simulink model "pid_position1"  (R2016b)
settings: Solver=VariableStepAuto  StartTime=0.0  StopTime=1  RelTol=1e-3
values from neighbouring files (symbols this model uses):
  Kd = -(1/(num(2,3)+num(2,4))*(poles(1)+poles(2)+poles(3))+den(1,2)/(num(2,3)+num(2,4)))*pi/180    [position1.m]    (also in position2.m = (1/(num(2,3)+num(2,4))*(poles(1)+poles(2)+poles(3))+den(1,2))
  Kd_p = 0    [position1.m]    (also in position2.m = 4.87)
  Ki = -(1/(num(2,3)+num(2,4))*(poles(1)*poles(2)*poles(3))+den(1,4)/(num(2,3)+num(2,4)))*pi/180    [position1.m]    (also in position2.m = (1/(num(2,3)+num(2,4))*(poles(1)*poles(2)*poles(3))+den(1,4))
  Ki_p = 0    [position1.m]    (also in position2.m = 0.197)
  Kp = -(den(1,3)/(num(2,3)+num(2,4))-1/(num(2,3)+num(2,4))*(poles(1)*poles(2)+poles(1)*poles(3)+poles(2)*poles(3)))*pi/180    [position1.m]    (also in position2.m = (den(1,3)/(num(2,3)+num(2,4))-1/(num(2,3)+num(2,4))*(poles(1)
  Kp_p = 16.8    [position1.m]    (also in position2.m = 1.96)
undefined symbols (not defined in the file or in its folder): den, num
settings Model: Creator=Ernie  LastModifiedBy=Ernie

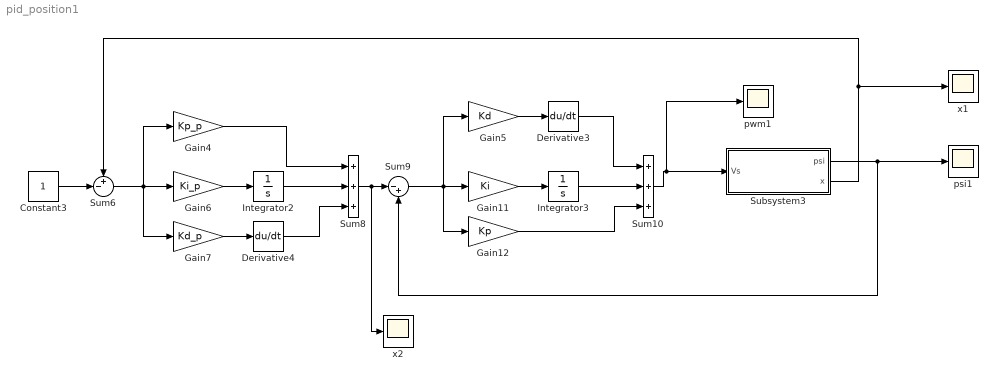
== system pid_position1 ==
  Constant3 : Constant
  Derivative3 : Derivative
  Derivative4 : Derivative
  Gain11 : Gain  Gain=Ki
  Gain12 : Gain  Gain=Kp
  Gain4 : Gain  Gain=Kp_p
  Gain5 : Gain  Gain=Kd
  Gain6 : Gain  Gain=Ki_p
  Gain7 : Gain  Gain=Kd_p
  Integrator2 : Integrator
  Integrator3 : Integrator
  Subsystem3 : Subsystem
  Sum10 : Sum  Inputs=+++
  Sum6 : Sum  Inputs=+-|
  Sum8 : Sum  Inputs=+++
  Sum9 : Sum  Inputs=|-+
  psi1 : Scope
  pwm1 : Scope
  x1 : Scope
  x2 : Scope
  wires:
  Sum8/1 -> x2/1, Sum9/1
  Gain11/1 -> Integrator3/1
  Integrator3/1 -> Sum10/2
  Gain12/1 -> Sum10/3
  Derivative3/1 -> Sum10/1
  Gain5/1 -> Derivative3/1
  Sum9/1 -> Gain5/1, Gain12/1, Gain11/1
  Subsystem3/1(psi) -> psi1/1, Sum9/2
  Constant3/1 -> Sum6/2
  Subsystem3/2(x) -> Sum6/1, x1/1
  Sum6/1 -> Gain7/1, Gain6/1, Gain4/1
  Gain7/1 -> Derivative4/1
  Gain6/1 -> Integrator2/1
  Derivative4/1 -> Sum8/3
  Integrator2/1 -> Sum8/2
  Gain4/1 -> Sum8/1
  Sum10/1 -> Subsystem3/1(Vs), pwm1/1

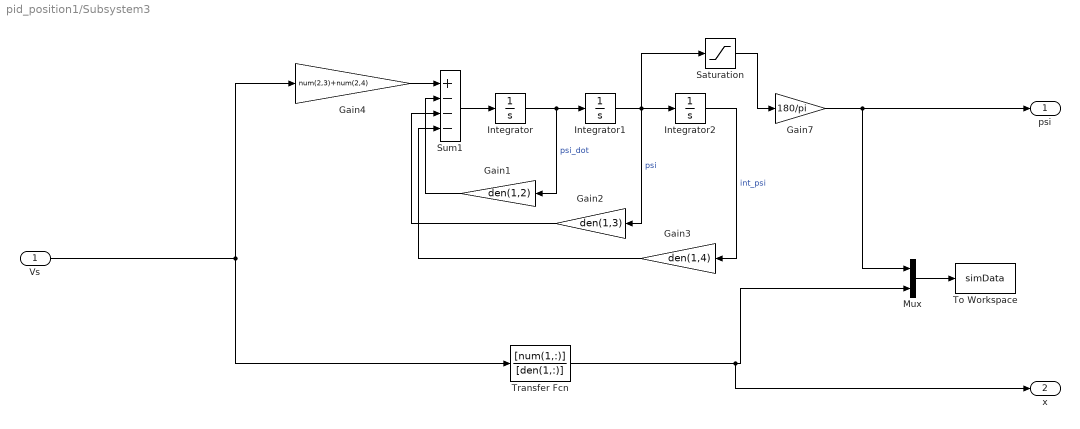
== system pid_position1/Subsystem3 ==
  Vs : Inport
  Gain1 : Gain  Gain=den(1,2)
  Gain2 : Gain  Gain=den(1,3)
  Gain3 : Gain  Gain=den(1,4)
  Gain4 : Gain  Gain=num(2,3)+num(2,4)
  Gain7 : Gain  Gain=180/pi
  Integrator : Integrator
  Integrator1 : Integrator  InitialCondition=10*pi/180
  Integrator2 : Integrator
  Mux : Mux  Inputs=2
  Saturation : Saturate  UpperLimit=pi/2  LowerLimit=-pi/2
  Sum1 : Sum  Inputs=+---
  To Workspace : ToWorkspace  VariableName=simData  SaveFormat=Timeseries  SampleTime=-1
  Transfer Fcn : TransferFcn  Numerator=[num(1,:)]  Denominator=[den(1,:)]
  psi : Outport
  x : Outport  Port=2
  wires:
  Mux/1 -> To Workspace/1
  Gain7/1 -> Mux/1, psi/1
  Integrator/1 -> Gain1/1, Integrator1/1  "psi_dot"
  Integrator1/1 -> Saturation/1, Gain2/1, Integrator2/1  "psi"
  Sum1/1 -> Integrator/1
  Gain1/1 -> Sum1/2
  Gain2/1 -> Sum1/3
  Integrator2/1 -> Gain3/1  "int_psi"
  Gain3/1 -> Sum1/4
  Gain4/1 -> Sum1/1
  Saturation/1 -> Gain7/1
  Transfer Fcn/1 -> x/1, Mux/2
  Vs/1 -> Transfer Fcn/1, Gain4/1
